simulink model "DataWeather"  (R2020b)
settings: configuration reference "GlobalConfig" (kept outside this file)
PreLoadFcn:
  | modelPreLoadClbck
InitFcn:
  | modelPreLoadClbck
settings Model: SimulationMode=accelerator  Creator=Oleg_2  LastModifiedBy=ofcra
settings ConfigSetRef: SourceName=GlobalConfig  SourceLocation=Base Workspace

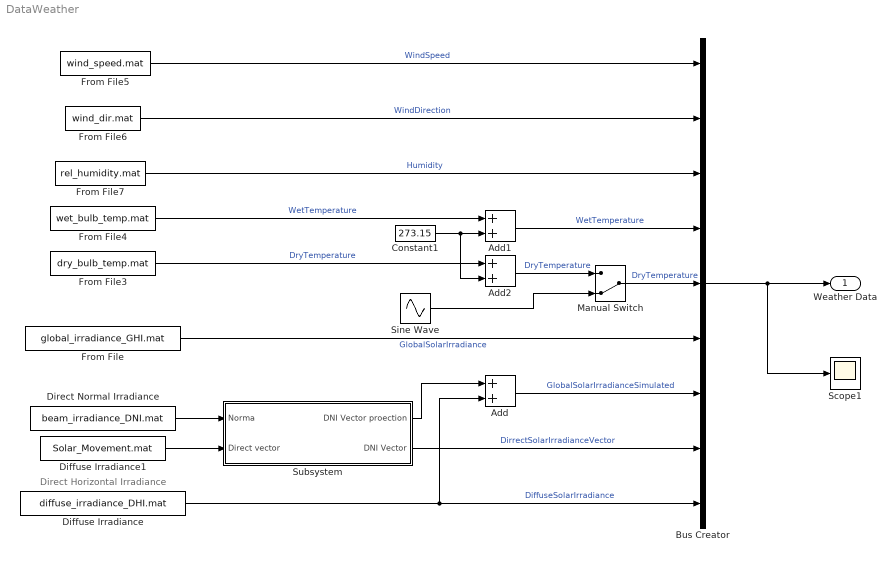
== system DataWeather ==
  note: Direct Horizontal Irradiance
  Add : Sum
  Add1 : Sum
  Add2 : Sum
  Bus Creator : BusCreator  Inputs=9  OutDataTypeStr=Bus: WeatherData
      settings: InheritFromInputs=off
  Constant1 : Constant  Value=273.15  OutDataTypeStr=double
  Diffuse Irradiance : FromFile  FileName=diffuse_irradiance_DHI.mat  OutDataTypeStr=double  ExtrapolationBeforeFirstDataPoint=Hold first value  ExtrapolationAfterLastDataPoint=Hold last value
  Diffuse Irradiance1 : FromFile  FileName=Solar_Movement.mat  OutDataTypeStr=double  ExtrapolationBeforeFirstDataPoint=Hold first value  ExtrapolationAfterLastDataPoint=Hold last value
  Direct Normal Irradiance : FromFile  FileName=beam_irradiance_DNI.mat  OutDataTypeStr=double  ExtrapolationBeforeFirstDataPoint=Hold first value  ExtrapolationAfterLastDataPoint=Hold last value
  From File : FromFile  FileName=global_irradiance_GHI.mat  OutDataTypeStr=double  ExtrapolationBeforeFirstDataPoint=Hold first value  ExtrapolationAfterLastDataPoint=Hold last value
  From File3 : FromFile  FileName=dry_bulb_temp.mat  OutDataTypeStr=double  ExtrapolationBeforeFirstDataPoint=Hold first value  ExtrapolationAfterLastDataPoint=Hold last value
  From File4 : FromFile  FileName=wet_bulb_temp.mat  OutDataTypeStr=double  ExtrapolationBeforeFirstDataPoint=Hold first value  ExtrapolationAfterLastDataPoint=Hold last value
  From File5 : FromFile  FileName=wind_speed.mat  OutDataTypeStr=double  ExtrapolationBeforeFirstDataPoint=Hold first value  ExtrapolationAfterLastDataPoint=Hold last value
  From File6 : FromFile  FileName=wind_dir.mat  OutDataTypeStr=double  ExtrapolationBeforeFirstDataPoint=Hold first value  ExtrapolationAfterLastDataPoint=Hold last value
  From File7 : FromFile  FileName=rel_humidity.mat  OutDataTypeStr=double  ExtrapolationBeforeFirstDataPoint=Hold first value  ExtrapolationAfterLastDataPoint=Hold last value
  Manual Switch : ManualSwitch  CurrentSetting=0
  Scope1 : Scope
  Sine Wave : Sin  Amplitude=12  Bias=13  Frequency=2*pi /3600 / 24/365  SampleTime=0
  Subsystem : Subsystem
  Weather Data : Outport  OutDataTypeStr=Bus: WeatherData
  wires:
  From File7/1 -> Bus Creator/3  "Humidity"
  From File6/1 -> Bus Creator/2  "WindDirection"
  From File5/1 -> Bus Creator/1  "WindSpeed"
  Add1/1 -> Bus Creator/4  "WetTemperature"
  Manual Switch/1 -> Bus Creator/5  "DryTemperature"
  From File/1 -> Bus Creator/6  "GlobalSolarIrradiance"
  Direct Normal Irradiance/1 -> Subsystem/1(Norma)
  Diffuse Irradiance/1 -> Bus Creator/9, Add/2  "DiffuseSolarIrradiance"
  Subsystem/2(DNI Vector) -> Bus Creator/8  "DirrectSolarIrradianceVector"
  Diffuse Irradiance1/1 -> Subsystem/2(Direct vector)
  Subsystem/1(DNI Vector proection) -> Add/1
  Add/1 -> Bus Creator/7  "GlobalSolarIrradianceSimulated"
  Bus Creator/1 -> Scope1/1, Weather Data/1
  From File4/1 -> Add1/1  "WetTemperature"
  From File3/1 -> Add2/1  "DryTemperature"
  Constant1/1 -> Add2/2, Add1/2
  Sine Wave/1 -> Manual Switch/2
  Add2/1 -> Manual Switch/1  "DryTemperature"

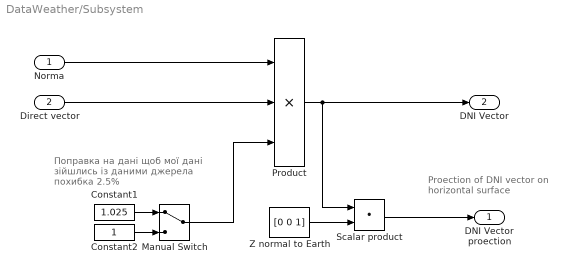
== system DataWeather/Subsystem ==
  note: Proection of DNI vector on
      |  horizontal surface
  note: Поправка на дані щоб мої дані
      | зійшлись із даними джерела
      | похибка 2.5%
  Norma : Inport
  Direct vector : Inport  Port=2
  Constant1 : Constant  Value=1.025  OutDataTypeStr=double
  Constant2 : Constant  OutDataTypeStr=double
  Manual Switch : ManualSwitch
  Product : Product  Inputs=3
  Scalar product : DotProduct  InputSameDT=on  OutDataTypeStr=Inherit: Inherit via internal rule
  Z normal to Earth : Constant  Value=[0 0 1]  OutDataTypeStr=double
  DNI Vector proection : Outport
  DNI Vector : Outport  Port=2
  wires:
  Constant2/1 -> Manual Switch/2
  Direct vector/1 -> Product/2
  Norma/1 -> Product/1
  Manual Switch/1 -> Product/3
  Constant1/1 -> Manual Switch/1
  Z normal to Earth/1 -> Scalar product/2
  Scalar product/1 -> DNI Vector proection/1
  Product/1 -> Scalar product/1, DNI Vector/1
